simulink model "MPS_device_passive"  (R2018b)
settings: Solver=ode4  StartTime=0  StopTime=700  FixedStep=0.02  MaxStep=0.02  RelTol=1e-3  EnableMultiTasking=on
InitFcn:
  | %SSModel_calc
undefined symbols (not defined in the file): body, CentralPTOPreload, constraint, L, ML1Preload, ML2Preload, ML3Preload, ML4Preload, ML5Preload, ML6Preload, ML7Preload, ML8Preload, mrelative, pto, PTOrotation, SidePTO1Preload, SidePTO2Preload, SidePTO3Preload, SidePTO4Preload, simu, waves, X, Y, Z
libraries: nesl_utility x580, sm_lib x317, vrlib x72, WECSim_Lib x36
(part 18 of 27)

== system MPS_device_passive/PTO P3F3/VisuP3F2/Hydrodynamic Body/Wave Diffraction and Excitation Force Calculation/Linear Wave Excitation Force Variant Subsystem/Regular Wave Excitation Force ==
  note: Calculates the wave force, F_wave, for the case of Regular Waves.
      |
      | F_wave =   A * cos(w * t) * Re{Fext}
      |                -  A * sin(w * t) * Im{Fext}
  In1 : Inport
  Add : Sum
  Add1 : Sum  Inputs=+-
  Constant : Constant  Value=pi/2
  Excitation Imaginary Part : Constant  Value=body.hydroForce.fExt.im(1,:)  VectorParams1D=off
  Excitation Real Part : Constant  Value=body.hydroForce.fExt.re(1,:)  VectorParams1D=off
  Product : Product
  Product1 : Product  Inputs=3
  Product2 : Product  Inputs=3
  Sine Wave Function : Sin  TimeSource=Use external signal  SampleTime=0
  Sine Wave Function1 : Sin  TimeSource=Use external signal  SampleTime=0
  Wave Amplitude : Constant  Value=waves.A(1,:)
  Wave Frequency : Constant  Value=waves.w(1,:)
  Out1 : Outport
  wires:
  Constant/1 -> Add/2
  Add/1 -> Sine Wave Function1/1
  Wave Amplitude/1 -> Product1/1, Product2/1  "A"
  Add1/1 -> Out1/1
  Product2/1 -> Add1/2
  Product1/1 -> Add1/1
  Excitation Real Part/1 -> Product1/2  "Re{Fext}"
  Excitation Imaginary Part/1 -> Product2/3  "Im{Fext}"
  Sine Wave Function/1 -> Product2/2  "sin(wt)"
  Sine Wave Function1/1 -> Product1/3  "cos(w*t)"
  Product/1 -> Add/1, Sine Wave Function/1
  Wave Frequency/1 -> Product/2  "w"
  In1/1 -> Product/1  "t"

== system MPS_device_passive/PTO P3F3/VisuP3F2/Hydrodynamic Body/Wave Diffraction and Excitation Force Calculation/Linear Wave Excitation Force Variant Subsystem/User Defined Wave Excitation Force ==
  note: Calculates the wave force, F_wave, for the case of User Defined Waves.
      |
      | F_wave = convolution calculation [1x6]
  InputWaveForceTimeHistory : FromWorkspace  VariableName=[waves.waveAmpTime(:,1),body.hydroForce.userDefinedFe]  SampleTime=0
  Out1 : Outport
  wires:
  InputWaveForceTimeHistory/1 -> Out1/1

== system MPS_device_passive/PTO P3F3/VisuP3F2/Hydrodynamic Body/Wave Diffraction and Excitation Force Calculation/Nonlinear FK Force Variant Subsystem/No Nonlinear FroudeKrylov Force ==
  Constant : Constant  Value=[0 0 0 0 0 0]
  Out1 : Outport
  wires:
  Constant/1 -> Out1/1

== system MPS_device_passive/PTO P3F3/VisuP3F2/Hydrodynamic Body/Wave Diffraction and Excitation Force Calculation/Nonlinear FK Force Variant Subsystem/With Nonlinear FroudeKrylov Force ==
  In1 : Inport
  In2 : Inport  Port=2
  In3 : Inport  Port=3
  Add : Sum  Inputs=+-
  Center of Gravity : Constant  Value=body.hydroData.properties.cg
  Center of Gravity1 : Constant  Value=body.hydroData.properties.cg
  Constant : Constant  Value=[0 0 0]
  Deep Water Flag : Constant  Value=waves.deepWaterWave
  Diffraction and Excitation Forces : MATLAB Function  TreatAsAtomicUnit=on
  Frequency Spacing : Constant  Value=waves.dw
  Gravity : Constant  Value=simu.g
  Mux : Mux  Inputs=2
  STL Areas : Constant  Value=body.bodyGeometry.area
  STL Centers : Constant  Value=body.bodyGeometry.center
  STL Normal Vectors : Constant  Value=body.bodyGeometry.norm
  To Workspace : ToWorkspace  VariableName=body13_wavenonlinearpressure_out  SaveFormat=Structure With Time  SampleTime=-1
      settings: Decimation=round(simu.dtOut/simu.dt,0)
  To Workspace1 : ToWorkspace  VariableName=body13_wavelinearpressure_out  SaveFormat=Structure With Time  SampleTime=-1
      settings: Decimation=round(simu.dtOut/simu.dt,0)
  Water Density : Constant  Value=simu.rho
  Water Depth : Constant  Value=waves.waterDepth
  Wave Amplitude : Constant  Value=waves.A
  Wave Frequency : Constant  Value=waves.w
  Wave Number : Constant  Value=waves.k
  Wave Random Phase : Constant  Value=waves.phaseRand
  Wave Type Number : Constant  Value=waves.typeNum
  fe_calc_time : Constant  Value=simu.dtFeNonlin
  simulation_sample_time : Constant  Value=simu.dt
  Out1 : Outport
  wires:
  STL Areas/1 -> Diffraction and Excitation Forces/5(area)
  fe_calc_time/1 -> Diffraction and Excitation Forces/19(dtFe)
  simulation_sample_time/1 -> Diffraction and Excitation Forces/18(dt)
  Diffraction and Excitation Forces/2(wp) -> To Workspace/1
  Diffraction and Excitation Forces/3(wpMeanFS) -> To Workspace1/1
  In2/1 -> Add/1
  Constant/1 -> Mux/2
  Center of Gravity/1 -> Mux/1  "cg"
  Mux/1 -> Add/2
  Add/1 -> Diffraction and Excitation Forces/1(x)  "x_cg"
  Deep Water Flag/1 -> Diffraction and Excitation Forces/13(deepWaterWave)
  Wave Random Phase/1 -> Diffraction and Excitation Forces/17(phaseRand)
  Water Depth/1 -> Diffraction and Excitation Forces/12(wDepth)
  Wave Number/1 -> Diffraction and Excitation Forces/14(k)
  Wave Type Number/1 -> Diffraction and Excitation Forces/15(typeNum)
  Frequency Spacing/1 -> Diffraction and Excitation Forces/11(dw)
  Wave Frequency/1 -> Diffraction and Excitation Forces/10(w)
  Wave Amplitude/1 -> Diffraction and Excitation Forces/9(AH)
  In1/1 -> Diffraction and Excitation Forces/16(t)
  In3/1 -> Diffraction and Excitation Forces/2(elv)
  STL Centers/1 -> Diffraction and Excitation Forces/3(center)
  STL Normal Vectors/1 -> Diffraction and Excitation Forces/4(tnorm)
  Water Density/1 -> Diffraction and Excitation Forces/6(rho)
  Gravity/1 -> Diffraction and Excitation Forces/7(g)
  Diffraction and Excitation Forces/1(f) -> Out1/1
  Center of Gravity1/1 -> Diffraction and Excitation Forces/8(cg)

== system MPS_device_passive/PTO P3F3/VisuP3F2/Hydrodynamic Body/Wave Radiation Forces Calculation/SS CI and Constant-Damping-CoeVariant Subsystem/Constant Coefficients ==
  In1 : Inport
  Product : Product  Multiplication=Matrix(*)
  Radiation Damping Matrix : Constant  Value=body.hydroForce.fDamping
  Out1 : Outport
  wires:
  In1/1 -> Product/2
  Product/1 -> Out1/1  "F_Single Frequency"
  Radiation Damping Matrix/1 -> Product/1

== system MPS_device_passive/PTO P3F3/VisuP3F2/Hydrodynamic Body/Wave Radiation Forces Calculation/SS CI and Constant-Damping-CoeVariant Subsystem/Convolution Integral Calculation ==
  In1 : Inport
  In2 : Inport  Port=2
  Body-to-Body Interactions Flag : Constant  Value=body.lenJ
  Fluid Memory : MATLAB Function  TreatAsAtomicUnit=on
  Impulse Response Function K : Constant  Value=body.hydroForce.irkb
  Time (relative to the current time step) : Constant  Value=simu.CTTime  SampleTime=simu.dt
  Out1 : Outport
  wires:
  In2/1 -> Fluid Memory/5(clockTime)
  Time (relative to the current time step)/1 -> Fluid Memory/4(CTTime)
  Impulse Response Function K/1 -> Fluid Memory/3(IRKB)
  In1/1 -> Fluid Memory/2(v)
  Fluid Memory/1(F_FM) -> Out1/1  "F_Convolution Integral"
  Body-to-Body Interactions Flag/1 -> Fluid Memory/1(lenJ)

== system MPS_device_passive/PTO P3F3/VisuP3F2/Hydrodynamic Body/Wave Radiation Forces Calculation/SS CI and Constant-Damping-CoeVariant Subsystem/State-Space Calculation  ==
  In1 : Inport
  State-Space : StateSpace  A=body.hydroForce.ssRadf.A  B=body.hydroForce.ssRadf.B  C=body.hydroForce.ssRadf.C  D=body.hydroForce.ssRadf.D  InitialCondition=0
  Out1 : Outport
  wires:
  State-Space/1 -> Out1/1
  In1/1 -> State-Space/1  "x"

== system MPS_device_passive/PTO P4F4/VisuP4F1/Hydrodynamic Body/B2B Subsystem/B2B/CrossCoupling ==
  note: CrossCoupling block is updated by its mask initialization, which is only called on when a simulation is run. 'From' blocks are automatically created and connected based on the number of bodies in the simulation.
  BC1 : BusCreator  Inputs=2
  BC2 : BusCreator  Inputs=2
  vel : Outport
  acc : Outport  Port=2
  wires:
  [acc2] -> BC2/2
  [vel2] -> BC1/2
  BC2/1 -> acc/1
  BC1/1 -> vel/1
  [acc1] -> BC2/1
  [vel1] -> BC1/1

== system MPS_device_passive/PTO P4F4/VisuP4F1/Hydrodynamic Body/Hydrostatic Restoring Force Calculation/Linear and Nonlinear Restoring Force Variant Subsystem/Linear Hydrostatic Restoring Force  ==
  In1 : Inport
  Add1 : Sum  Inputs=+-
  Add2 : Sum
  Assignment (Add Net Bouyancy Force to Z-Direction) : Assignment  IndexOptions=Index vector (dialog)  Indices=3  OutputSizes=1
  Body Mass : Constant  Value=body.hydroForce.storage.mass
  Constant1 : Constant  Value=[0 0 0 0 0 0]
  Gravity : Constant  Value=simu.g
  Linear Restioring Coefficient Matrix : Constant  Value=body.hydroForce.linearHydroRestCoef
  Product : Product
  Product1 : Product  Inputs=3
  Product2 : Product  Multiplication=Matrix(*)
  Volume : Constant  Value=body.dispVol
  Water Density : Constant  Value=simu.rho
  Out1 : Outport
  wires:
  Linear Restioring Coefficient Matrix/1 -> Product2/1  "K"
  Product2/1 -> Add2/2  "Linear Restoring Force"
  Add1/1 -> Assignment (Add Net Bouyancy Force to Z-Direction)/2
  Product1/1 -> Add1/2  "F_Buoyancy"
  Product/1 -> Add1/1  "F_Gravity"
  Water Density/1 -> Product1/1  "rho"
  Gravity/1 -> Product/1, Product1/2  "g"
  Volume/1 -> Product1/3  "Vol"
  Add2/1 -> Out1/1  "F_Restoring"
  Assignment (Add Net Bouyancy Force to Z-Direction)/1 -> Add2/1  "Net Buoyancy Force"
  Constant1/1 -> Assignment (Add Net Bouyancy Force to Z-Direction)/1
  Body Mass/1 -> Product/2  "m"
  In1/1 -> Product2/2  "x"

== system MPS_device_passive/PTO P4F4/VisuP4F1/Hydrodynamic Body/Hydrostatic Restoring Force Calculation/Linear and Nonlinear Restoring Force Variant Subsystem/Nonlinear Hydrostatic Restoring Force ==
  In1 : Inport
  In2 : Inport  Port=2
  In3 : Inport  Port=3
  Add3 : Sum  Inputs=-+
  Assignment (Add Net Bouyancy Force to Z-Direction)2 : Assignment  IndexOptions=Index vector (dialog)  Indices=3  OutputSizes=1
  Body Mass1 : Constant  Value=body.hydroForce.storage.mass
  Center of Gravity : Constant  Value=body.cg
  Constant2 : Constant  Value=[0 0 0 0 0 0]
  Diffarction and Excitation Forces1 : MATLAB Function  TreatAsAtomicUnit=on
  Gravity2 : Constant  Value=simu.g
  Product3 : Product
  SImulation Step Time : Constant  Value=simu.dt
  STL areas : Constant  Value=body.bodyGeometry.area
  STL centers : Constant  Value=body.bodyGeometry.center
  STL normal vectors : Constant  Value=body.bodyGeometry.norm
  Simulation Fe Calc Step Time : Constant  Value=simu.dtFeNonlin
  To Workspace1 : ToWorkspace  VariableName=body16_hspressure_out  SaveFormat=Structure With Time  SampleTime=-1
      settings: Decimation=round(simu.dtOut/simu.dt,0)
  Water Density1 : Constant  Value=simu.rho
  Out1 : Outport
  wires:
  STL areas/1 -> Diffarction and Excitation Forces1/5(area)
  In3/1 -> Diffarction and Excitation Forces1/11(t)
  Simulation Fe Calc Step Time/1 -> Diffarction and Excitation Forces1/10(dtFe)
  SImulation Step Time/1 -> Diffarction and Excitation Forces1/9(dt)
  Diffarction and Excitation Forces1/2(p) -> To Workspace1/1
  In2/1 -> Diffarction and Excitation Forces1/2(elv)
  STL centers/1 -> Diffarction and Excitation Forces1/3(center)
  STL normal vectors/1 -> Diffarction and Excitation Forces1/4(tnorm)
  Water Density1/1 -> Diffarction and Excitation Forces1/6(rho)
  Gravity2/1 -> Diffarction and Excitation Forces1/7(g), Product3/1  "g"
  Body Mass1/1 -> Product3/2
  Constant2/1 -> Assignment (Add Net Bouyancy Force to Z-Direction)2/1
  Product3/1 -> Assignment (Add Net Bouyancy Force to Z-Direction)2/2
  Diffarction and Excitation Forces1/1(f) -> Add3/1
  Add3/1 -> Out1/1
  Assignment (Add Net Bouyancy Force to Z-Direction)2/1 -> Add3/2
  Center of Gravity/1 -> Diffarction and Excitation Forces1/8(cg)
  In1/1 -> Diffarction and Excitation Forces1/1(x)

== system MPS_device_passive/PTO P4F4/VisuP4F1/Hydrodynamic Body/Morrison Element and ViscousDampingForceCalculation/Morrison Element Variant Subsystem/Morrison Element Off ==
  Constant : Constant  Value=[0 0 0 0 0 0]
  morison_force : Outport
  wires:
  Constant/1 -> morison_force/1

== system MPS_device_passive/PTO P4F4/VisuP4F1/Hydrodynamic Body/Morrison Element and ViscousDampingForceCalculation/Morrison Element Variant Subsystem/Morrison Element On ==
  note: 1) Add Subsystem or Model blocks as valid variant choices.
      | 2) You cannot connect blocks at this level. At simulation, connectivity is automatically
      | determined, based on the active variant and port name matching.
  displacement : Inport
  velocity : Inport  Port=2
  acceleration : Inport  Port=3
  time : Inport  Port=4
  Irregular Wave Morison Force : Subsystem  VariantControl=sv_irregularWaves
  No Wave Morison Force : Subsystem  VariantControl=sv_noWave
  Regular Wave Morison Force : Subsystem  VariantControl=sv_regularWaves
  morison_force : Outport

== system MPS_device_passive/PTO P4F4/VisuP4F1/Hydrodynamic Body/Nonlinear Wave Elevation/Linear or Instantaneous Free Surface/Instantaneous Water Free Surface   ==
  In1 : Inport
  In2 : Inport  Port=2
  Center of Gravity : Constant  Value=body.cg
  Frequency Spacing : Constant  Value=waves.dw
  Instantaneous FS : MATLAB Function  TreatAsAtomicUnit=on
  Ramp Time : Constant  Value=simu.rampT
  STL Centers : Constant  Value=body.bodyGeometry.center
  Simulation Time Step : Constant  Value=simu.dt
  Time Step for Non-Linear Forces : Constant  Value=simu.dtFeNonlin
  Wave Amplitude : Constant  Value=waves.A
  Wave Direction : Constant  Value=waves.waveDir
  Wave Frequency : Constant  Value=waves.w
  Wave Number : Constant  Value=waves.k
  Wave Random Phase : Constant  Value=waves.phaseRand
  Wave Type Number : Constant  Value=waves.typeNum
  Out1 : Outport
  wires:
  Wave Amplitude/1 -> Instantaneous FS/4(AH)
  Time Step for Non-Linear Forces/1 -> Instantaneous FS/14(dtFe)
  Simulation Time Step/1 -> Instantaneous FS/13(dt)
  Wave Direction/1 -> Instantaneous FS/12(waveDir)
  In1/1 -> Instantaneous FS/1(x)
  In2/1 -> Instantaneous FS/9(t)
  Frequency Spacing/1 -> Instantaneous FS/6(dw)
  Wave Random Phase/1 -> Instantaneous FS/11(phaseRand)
  Ramp Time/1 -> Instantaneous FS/10(rampT)
  Wave Type Number/1 -> Instantaneous FS/8(typeNum)
  Wave Frequency/1 -> Instantaneous FS/5(w)
  Wave Number/1 -> Instantaneous FS/7(k)
  Center of Gravity/1 -> Instantaneous FS/3(cg)
  STL Centers/1 -> Instantaneous FS/2(center)
  Instantaneous FS/1(f) -> Out1/1

== system MPS_device_passive/PTO P4F4/VisuP4F1/Hydrodynamic Body/Nonlinear Wave Elevation/Linear or Instantaneous Free Surface/Mean Water Free Surface  ==
  zero : Constant  Value=0
  Out1 : Outport
  wires:
  zero/1 -> Out1/1

== system MPS_device_passive/PTO P4F4/VisuP4F1/Hydrodynamic Body/Wave Diffraction and Excitation Force Calculation/Linear Wave Excitation Force Variant Subsystem/Irregular Wave Excitation Force ==
  note: Calculates the wave force, F_wave, for the case of Irregular Waves.
      |
      | F_wave = sum( F_wave(i))
      |
      | where i = each frequency bin.
  In1 : Inport
  Frequency Spacing Delta Omega : Constant  Value=waves.dw  VectorParams1D=off
  Imaginary Part of Wave Excitation : Constant  Value=body.hydroForce.fExt.im  VectorParams1D=off
  MATLAB Function : MATLAB Function  TreatAsAtomicUnit=on
  Random Phase : Constant  Value=waves.phaseRand  VectorParams1D=off
  Real Part of Wave Excitation : Constant  Value=body.hydroForce.fExt.re  VectorParams1D=off
  Wave Frequency : Constant  Value=waves.w  VectorParams1D=off
  Wave Spectrum : Constant  Value=waves.A  VectorParams1D=off
  Out1 : Outport
  wires:
  Frequency Spacing Delta Omega/1 -> MATLAB Function/6(dw)
  In1/1 -> MATLAB Function/7(time)
  Wave Spectrum/1 -> MATLAB Function/1(A)
  Real Part of Wave Excitation/1 -> MATLAB Function/3(fExtRE)
  Imaginary Part of Wave Excitation/1 -> MATLAB Function/4(fExtIM)
  Wave Frequency/1 -> MATLAB Function/2(w)
  MATLAB Function/1(Fext) -> Out1/1
  Random Phase/1 -> MATLAB Function/5(phaseRand)

== system MPS_device_passive/PTO P4F4/VisuP4F1/Hydrodynamic Body/Wave Diffraction and Excitation Force Calculation/Linear Wave Excitation Force Variant Subsystem/No Wave Excitation Force ==
  Constant : Constant  Value=[0 0 0 0 0 0]
  Out1 : Outport
  wires:
  Constant/1 -> Out1/1

== system MPS_device_passive/PTO P4F4/VisuP4F1/Hydrodynamic Body/Wave Diffraction and Excitation Force Calculation/Linear Wave Excitation Force Variant Subsystem/Regular Wave Excitation Force ==
  note: Calculates the wave force, F_wave, for the case of Regular Waves.
      |
      | F_wave =   A * cos(w * t) * Re{Fext}
      |                -  A * sin(w * t) * Im{Fext}
  In1 : Inport
  Add : Sum
  Add1 : Sum  Inputs=+-
  Constant : Constant  Value=pi/2
  Excitation Imaginary Part : Constant  Value=body.hydroForce.fExt.im(1,:)  VectorParams1D=off
  Excitation Real Part : Constant  Value=body.hydroForce.fExt.re(1,:)  VectorParams1D=off
  Product : Product
  Product1 : Product  Inputs=3
  Product2 : Product  Inputs=3
  Sine Wave Function : Sin  TimeSource=Use external signal  SampleTime=0
  Sine Wave Function1 : Sin  TimeSource=Use external signal  SampleTime=0
  Wave Amplitude : Constant  Value=waves.A(1,:)
  Wave Frequency : Constant  Value=waves.w(1,:)
  Out1 : Outport
  wires:
  Constant/1 -> Add/2
  Add/1 -> Sine Wave Function1/1
  Wave Amplitude/1 -> Product1/1, Product2/1  "A"
  Add1/1 -> Out1/1
  Product2/1 -> Add1/2
  Product1/1 -> Add1/1
  Excitation Real Part/1 -> Product1/2  "Re{Fext}"
  Excitation Imaginary Part/1 -> Product2/3  "Im{Fext}"
  Sine Wave Function/1 -> Product2/2  "sin(wt)"
  Sine Wave Function1/1 -> Product1/3  "cos(w*t)"
  Product/1 -> Add/1, Sine Wave Function/1
  Wave Frequency/1 -> Product/2  "w"
  In1/1 -> Product/1  "t"

== system MPS_device_passive/PTO P4F4/VisuP4F1/Hydrodynamic Body/Wave Diffraction and Excitation Force Calculation/Linear Wave Excitation Force Variant Subsystem/User Defined Wave Excitation Force ==
  note: Calculates the wave force, F_wave, for the case of User Defined Waves.
      |
      | F_wave = convolution calculation [1x6]
  InputWaveForceTimeHistory : FromWorkspace  VariableName=[waves.waveAmpTime(:,1),body.hydroForce.userDefinedFe]  SampleTime=0
  Out1 : Outport
  wires:
  InputWaveForceTimeHistory/1 -> Out1/1

== system MPS_device_passive/PTO P4F4/VisuP4F1/Hydrodynamic Body/Wave Diffraction and Excitation Force Calculation/Nonlinear FK Force Variant Subsystem/No Nonlinear FroudeKrylov Force ==
  Constant : Constant  Value=[0 0 0 0 0 0]
  Out1 : Outport
  wires:
  Constant/1 -> Out1/1

== system MPS_device_passive/PTO P4F4/VisuP4F1/Hydrodynamic Body/Wave Diffraction and Excitation Force Calculation/Nonlinear FK Force Variant Subsystem/With Nonlinear FroudeKrylov Force ==
  In1 : Inport
  In2 : Inport  Port=2
  In3 : Inport  Port=3
  Add : Sum  Inputs=+-
  Center of Gravity : Constant  Value=body.hydroData.properties.cg
  Center of Gravity1 : Constant  Value=body.hydroData.properties.cg
  Constant : Constant  Value=[0 0 0]
  Deep Water Flag : Constant  Value=waves.deepWaterWave
  Diffraction and Excitation Forces : MATLAB Function  TreatAsAtomicUnit=on
  Frequency Spacing : Constant  Value=waves.dw
  Gravity : Constant  Value=simu.g
  Mux : Mux  Inputs=2
  STL Areas : Constant  Value=body.bodyGeometry.area
  STL Centers : Constant  Value=body.bodyGeometry.center
  STL Normal Vectors : Constant  Value=body.bodyGeometry.norm
  To Workspace : ToWorkspace  VariableName=body16_wavenonlinearpressure_out  SaveFormat=Structure With Time  SampleTime=-1
      settings: Decimation=round(simu.dtOut/simu.dt,0)
  To Workspace1 : ToWorkspace  VariableName=body16_wavelinearpressure_out  SaveFormat=Structure With Time  SampleTime=-1
      settings: Decimation=round(simu.dtOut/simu.dt,0)
  Water Density : Constant  Value=simu.rho
  Water Depth : Constant  Value=waves.waterDepth
  Wave Amplitude : Constant  Value=waves.A
  Wave Frequency : Constant  Value=waves.w
  Wave Number : Constant  Value=waves.k
  Wave Random Phase : Constant  Value=waves.phaseRand
  Wave Type Number : Constant  Value=waves.typeNum
  fe_calc_time : Constant  Value=simu.dtFeNonlin
  simulation_sample_time : Constant  Value=simu.dt
  Out1 : Outport
  wires:
  STL Areas/1 -> Diffraction and Excitation Forces/5(area)
  fe_calc_time/1 -> Diffraction and Excitation Forces/19(dtFe)
  simulation_sample_time/1 -> Diffraction and Excitation Forces/18(dt)
  Diffraction and Excitation Forces/2(wp) -> To Workspace/1
  Diffraction and Excitation Forces/3(wpMeanFS) -> To Workspace1/1
  In2/1 -> Add/1
  Constant/1 -> Mux/2
  Center of Gravity/1 -> Mux/1  "cg"
  Mux/1 -> Add/2
  Add/1 -> Diffraction and Excitation Forces/1(x)  "x_cg"
  Deep Water Flag/1 -> Diffraction and Excitation Forces/13(deepWaterWave)
  Wave Random Phase/1 -> Diffraction and Excitation Forces/17(phaseRand)
  Water Depth/1 -> Diffraction and Excitation Forces/12(wDepth)
  Wave Number/1 -> Diffraction and Excitation Forces/14(k)
  Wave Type Number/1 -> Diffraction and Excitation Forces/15(typeNum)
  Frequency Spacing/1 -> Diffraction and Excitation Forces/11(dw)
  Wave Frequency/1 -> Diffraction and Excitation Forces/10(w)
  Wave Amplitude/1 -> Diffraction and Excitation Forces/9(AH)
  In1/1 -> Diffraction and Excitation Forces/16(t)
  In3/1 -> Diffraction and Excitation Forces/2(elv)
  STL Centers/1 -> Diffraction and Excitation Forces/3(center)
  STL Normal Vectors/1 -> Diffraction and Excitation Forces/4(tnorm)
  Water Density/1 -> Diffraction and Excitation Forces/6(rho)
  Gravity/1 -> Diffraction and Excitation Forces/7(g)
  Diffraction and Excitation Forces/1(f) -> Out1/1
  Center of Gravity1/1 -> Diffraction and Excitation Forces/8(cg)

== system MPS_device_passive/PTO P4F4/VisuP4F1/Hydrodynamic Body/Wave Radiation Forces Calculation/SS CI and Constant-Damping-CoeVariant Subsystem/Constant Coefficients ==
  In1 : Inport
  Product : Product  Multiplication=Matrix(*)
  Radiation Damping Matrix : Constant  Value=body.hydroForce.fDamping
  Out1 : Outport
  wires:
  In1/1 -> Product/2
  Product/1 -> Out1/1  "F_Single Frequency"
  Radiation Damping Matrix/1 -> Product/1

== system MPS_device_passive/PTO P4F4/VisuP4F1/Hydrodynamic Body/Wave Radiation Forces Calculation/SS CI and Constant-Damping-CoeVariant Subsystem/Convolution Integral Calculation ==
  In1 : Inport
  In2 : Inport  Port=2
  Body-to-Body Interactions Flag : Constant  Value=body.lenJ
  Fluid Memory : MATLAB Function  TreatAsAtomicUnit=on
  Impulse Response Function K : Constant  Value=body.hydroForce.irkb
  Time (relative to the current time step) : Constant  Value=simu.CTTime  SampleTime=simu.dt
  Out1 : Outport
  wires:
  In2/1 -> Fluid Memory/5(clockTime)
  Time (relative to the current time step)/1 -> Fluid Memory/4(CTTime)
  Impulse Response Function K/1 -> Fluid Memory/3(IRKB)
  In1/1 -> Fluid Memory/2(v)
  Fluid Memory/1(F_FM) -> Out1/1  "F_Convolution Integral"
  Body-to-Body Interactions Flag/1 -> Fluid Memory/1(lenJ)

== system MPS_device_passive/PTO P4F4/VisuP4F1/Hydrodynamic Body/Wave Radiation Forces Calculation/SS CI and Constant-Damping-CoeVariant Subsystem/State-Space Calculation  ==
  In1 : Inport
  State-Space : StateSpace  A=body.hydroForce.ssRadf.A  B=body.hydroForce.ssRadf.B  C=body.hydroForce.ssRadf.C  D=body.hydroForce.ssRadf.D  InitialCondition=0
  Out1 : Outport
  wires:
  State-Space/1 -> Out1/1
  In1/1 -> State-Space/1  "x"

== system MPS_device_passive/Reactor/Hydrodynamic Body/Morrison Element and ViscousDampingForceCalculation/Morrison Element Variant Subsystem/Morrison Element On/Irregular Wave Excitation Force ==
  In1 : Inport
  In2 : Inport  Port=2
  In3 : Inport  Port=3
  In4 : Inport  Port=4
  Area : Constant  Value=body.morrisonElement.characteristicArea  VectorParams1D=off
  Ca : Constant  Value=body.morrisonElement.ca  VectorParams1D=off
  Cd : Constant  Value=body.morrisonElement.cd  VectorParams1D=off
  MESum : Sum  Inputs=+  CollapseMode=Specified dimension
  MorrisonElements : Subsystem  TreatAsAtomicUnit=on
  Reshape : Reshape
  Volume : Constant  Value=body.morrisonElement.VME  VectorParams1D=off
  "r_{g}" : Constant  Value=body.morrisonElement.rgME  VectorParams1D=off
  Out1 : Outport
  wires:
  In4/1 -> MorrisonElements/9(Time)
  MESum/1 -> Reshape/1
  Reshape/1 -> Out1/1
  MorrisonElements/1(Force) -> MESum/1
  Ca/1 -> MorrisonElements/8(Ca)
  Volume/1 -> MorrisonElements/7(Vol)
  In3/1 -> MorrisonElements/3(Accel)
  In1/1 -> MorrisonElements/4(Disp)
  Cd/1 -> MorrisonElements/6(Cd)
  Area/1 -> MorrisonElements/5(A)
  "r_{g}"/1 -> MorrisonElements/1(r)
  In2/1 -> MorrisonElements/2(Vel)

== system MPS_device_passive/Reactor/Hydrodynamic Body/Morrison Element and ViscousDampingForceCalculation/Morrison Element Variant Subsystem/Morrison Element On/No Wave Excitation Force ==
  In1 : Inport
  In2 : Inport  Port=2
  In3 : Inport  Port=3
  In4 : Inport  Port=4
  Area : Constant  Value=body.morrisonElement.characteristicArea  VectorParams1D=off
  Ca : Constant  Value=body.morrisonElement.ca  VectorParams1D=off
  Cd : Constant  Value=body.morrisonElement.cd  VectorParams1D=off
  MESum : Sum  Inputs=+  CollapseMode=Specified dimension
  MorrisonElements : Subsystem  TreatAsAtomicUnit=on
  Reshape : Reshape
  Volume : Constant  Value=body.morrisonElement.VME  VectorParams1D=off
  "r_{g}" : Constant  Value=body.morrisonElement.rgME  VectorParams1D=off
  Out1 : Outport
  wires:
  In4/1 -> MorrisonElements/9(Time)
  Reshape/1 -> Out1/1
  MESum/1 -> Reshape/1
  In3/1 -> MorrisonElements/3(Accel)
  In2/1 -> MorrisonElements/2(Vel)
  In1/1 -> MorrisonElements/4(Disp)
  Ca/1 -> MorrisonElements/8(Ca)
  Volume/1 -> MorrisonElements/7(Vol)
  MorrisonElements/1(Force) -> MESum/1
  Cd/1 -> MorrisonElements/6(Cd)
  Area/1 -> MorrisonElements/5(Area)
  "r_{g}"/1 -> MorrisonElements/1(r)

== system MPS_device_passive/Reactor/Hydrodynamic Body/Morrison Element and ViscousDampingForceCalculation/Morrison Element Variant Subsystem/Morrison Element On/Regular Wave Excitation Force ==
  In1 : Inport
  In2 : Inport  Port=2
  In3 : Inport  Port=3
  In4 : Inport  Port=4
  Area : Constant  Value=body.morrisonElement.characteristicArea  VectorParams1D=off
  Ca : Constant  Value=body.morrisonElement.ca  VectorParams1D=off
  Cd : Constant  Value=body.morrisonElement.cd  VectorParams1D=off
  MESum : Sum  Inputs=+  CollapseMode=Specified dimension
  MorrisonElements : Subsystem  TreatAsAtomicUnit=on
  Reshape : Reshape
  Volume : Constant  Value=body.morrisonElement.VME  VectorParams1D=off
  "r_{g}" : Constant  Value=body.morrisonElement.rgME  VectorParams1D=off
  Out1 : Outport
  wires:
  In4/1 -> MorrisonElements/9(Time)
  Reshape/1 -> Out1/1
  MESum/1 -> Reshape/1
  In3/1 -> MorrisonElements/3(Accel)
  In2/1 -> MorrisonElements/2(Vel)
  In1/1 -> MorrisonElements/4(Disp)
  Ca/1 -> MorrisonElements/8(Ca)
  Volume/1 -> MorrisonElements/7(Vol)
  MorrisonElements/1(Force) -> MESum/1
  Cd/1 -> MorrisonElements/6(Cd)
  Area/1 -> MorrisonElements/5(Area)
  "r_{g}"/1 -> MorrisonElements/1(r)

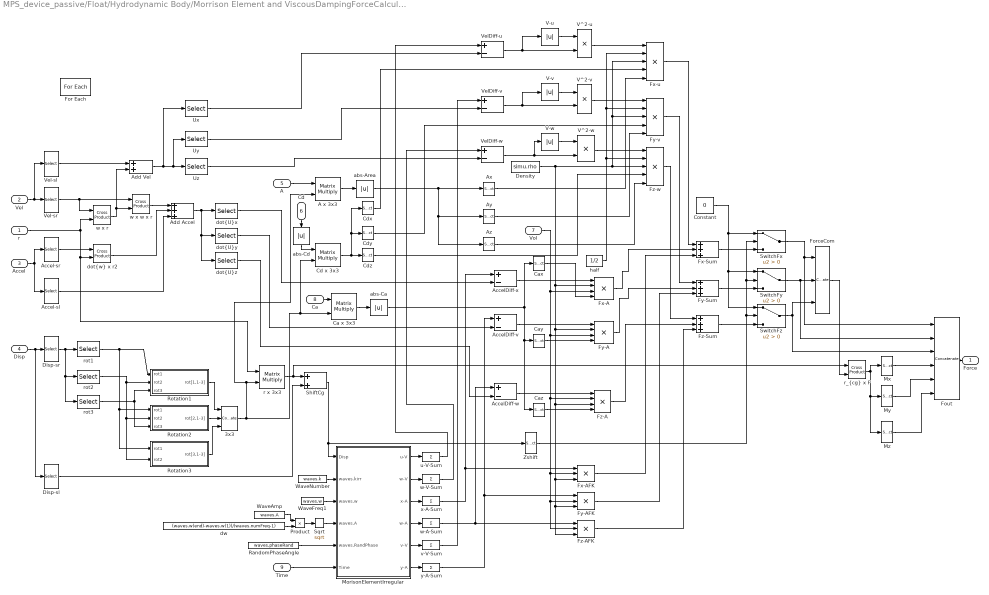
== system MPS_device_passive/Float/Hydrodynamic Body/Morrison Element and ViscousDampingForceCalculation/Morrison Element Variant Subsystem/Morrison Element On/Irregular Wave Morison Force/MorrisonElements ==
  r : Inport  Partition=on  PartitionDimension=1  PartitionWidth=1  PartitionOffset=0
  Vel : Inport  Port=2
  Accel : Inport  Port=3
  Disp : Inport  Port=4
  A : Inport  Port=5  Partition=on  PartitionDimension=1  PartitionWidth=1  PartitionOffset=0
  Cd : Inport  Port=6  Partition=on  PartitionDimension=1  PartitionWidth=1  PartitionOffset=0
  Vol : Inport  Port=7  Partition=on  PartitionDimension=1  PartitionWidth=1  PartitionOffset=0
  Ca : Inport  Port=8  Partition=on  PartitionDimension=1  PartitionWidth=1  PartitionOffset=0
  Time : Inport  Port=9
  3x3 : Concatenate  NumInputs=3  Mode=Multidimensional array
  A x 3x3 : Product  Multiplication=Matrix(*)
  Accel-sl : Selector  InputPortWidth=6  IndexOptions=Index vector (dialog)  Indices=[1 2 3]  OutputSizes=1
  Accel-sr : Selector  InputPortWidth=6  IndexOptions=Index vector (dialog)  Indices=[4 5 6]  OutputSizes=1
  AccelDiff-v : Sum  Inputs=+-
  AccelDiff-w : Sum  Inputs=+-
  AccelDiff-x : Sum  Inputs=+-
  Add Accel : Sum  Inputs=+++
  Add Vel : Sum
  Ax : Selector  InputPortWidth=3  IndexOptions=Index vector (dialog)  Indices=[1]  OutputSizes=1
  Ay : Selector  InputPortWidth=3  IndexOptions=Index vector (dialog)  Indices=[2]  OutputSizes=1
  Az : Selector  InputPortWidth=3  IndexOptions=Index vector (dialog)  Indices=[3]  OutputSizes=1
  Ca x 3x3 : Product  Multiplication=Matrix(*)
  Cax : Selector  InputPortWidth=3  IndexOptions=Index vector (dialog)  Indices=[1]  OutputSizes=1
  Cay : Selector  InputPortWidth=3  IndexOptions=Index vector (dialog)  Indices=[2]  OutputSizes=1
  Caz : Selector  InputPortWidth=3  IndexOptions=Index vector (dialog)  Indices=[3]  OutputSizes=1
  Cd x 3x3 : Product  Multiplication=Matrix(*)
  Cdx : Selector  InputPortWidth=3  IndexOptions=Index vector (dialog)  Indices=[1]  OutputSizes=1
  Cdy : Selector  InputPortWidth=3  IndexOptions=Index vector (dialog)  Indices=[2]  OutputSizes=1
  Cdz : Selector  InputPortWidth=3  IndexOptions=Index vector (dialog)  Indices=[3]  OutputSizes=1
  Constant : Constant  Value=0
  Density : Constant  Value=simu.rho
  Disp-sl : Selector  InputPortWidth=6  IndexOptions=Index vector (dialog)  Indices=[1 2 3]  OutputSizes=1
  Disp-sr : Selector  InputPortWidth=6  IndexOptions=Index vector (dialog)  Indices=[4 5 6]  OutputSizes=1
  For Each : ForEach  DisableCoverage=on  IndexMode=One-based
  ForceCom : Concatenate  NumInputs=3  ConcatenateDimension=2
  Fout : Concatenate  NumInputs=6  Mode=Multidimensional array  ConcatenateDimension=2
  Fx-A : Product  Inputs=4
  Fx-AFK : Product  Inputs=3
  Fx-Sum : Sum  Inputs=+++
  Fx-u : Product  Inputs=5
  Fy-A : Product  Inputs=4
  Fy-AFK : Product  Inputs=3
  Fy-Sum : Sum  Inputs=+++
  Fy-v : Product  Inputs=5
  Fz-A : Product  Inputs=4
  Fz-AFK : Product  Inputs=3
  Fz-Sum : Sum  Inputs=+++
  Fz-w : Product  Inputs=5
  MorisonElementIrregular : Subsystem  TreatAsAtomicUnit=on
  Mx : Selector  InputPortWidth=3  IndexOptions=Index vector (dialog)  Indices=[1]  OutputSizes=1
  My : Selector  InputPortWidth=3  IndexOptions=Index vector (dialog)  Indices=[2]  OutputSizes=1
  Mz : Selector  InputPortWidth=3  IndexOptions=Index vector (dialog)  Indices=[3]  OutputSizes=1
  Product : Product
  RandomPhaseAngle : Constant  Value=waves.phaseRand  VectorParams1D=off
  Rotation1 : Subsystem
  Rotation2 : Subsystem
  Rotation3 : Subsystem
  ShiftCg : Sum
  Sqrt : Sqrt  SaturateOnIntegerOverflow=on
  SwitchFx : Switch  Criteria=u2 > Threshold
  SwitchFy : Switch  Criteria=u2 > Threshold
  SwitchFz : Switch  Criteria=u2 > Threshold
  Ux : Selector  InputPortWidth=3  IndexOptions=Index vector (dialog)  Indices=[1]  OutputSizes=1
  Uy : Selector  InputPortWidth=3  IndexOptions=Index vector (dialog)  Indices=[2]  OutputSizes=1
  Uz : Selector  InputPortWidth=3  IndexOptions=Index vector (dialog)  Indices=[3]  OutputSizes=1
  V-u : Abs
  V-v : Abs
  V-w : Abs
  V^2-u : Product
  V^2-v : Product
  V^2-w : Product
  Vel-sl : Selector  InputPortWidth=6  IndexOptions=Index vector (dialog)  Indices=[1 2 3]  OutputSizes=1
  "Vel-sr " : Selector  InputPortWidth=6  IndexOptions=Index vector (dialog)  Indices=[4 5 6]  OutputSizes=1
  VelDiff-u : Sum  Inputs=+-
  VelDiff-v : Sum  Inputs=+-
  VelDiff-w : Sum  Inputs=+-
  WaveAmp : Constant  Value=waves.A  VectorParams1D=off
  WaveFreq1 : Constant  Value=waves.w  VectorParams1D=off
  WaveNumber : Constant  Value=waves.k  VectorParams1D=off
  Zshift : Selector  InputPortWidth=3  IndexOptions=Index vector (dialog)  Indices=[3]  OutputSizes=1
  abs-Area : Abs
  abs-Ca : Abs
  abs-Cd : Abs
  "dot{U}x" : Selector  InputPortWidth=3  IndexOptions=Index vector (dialog)  Indices=[1]  OutputSizes=1
  "dot{U}y" : Selector  InputPortWidth=3  IndexOptions=Index vector (dialog)  Indices=[2]  OutputSizes=1
  "dot{U}z" : Selector  InputPortWidth=3  IndexOptions=Index vector (dialog)  Indices=[3]  OutputSizes=1
  "dot{w} x r2" : vrlib/Utilities/Cross Product
      settings: SourceProductBaseCode=VR
  dw : Constant  Value=(waves.w(end)-waves.w(1))/(waves.numFreq-1)  VectorParams1D=off
  half : Constant  Value=1/2
  r x 3x3 : Product  Multiplication=Matrix(*)
  "r_{cg} x F" : vrlib/Utilities/Cross Product
      settings: SourceProductBaseCode=VR
  rot1 : Selector  InputPortWidth=3  IndexOptions=Index vector (dialog)  Indices=[1]  OutputSizes=1
  rot2 : Selector  InputPortWidth=3  IndexOptions=Index vector (dialog)  Indices=[2]  OutputSizes=1
  rot3 : Selector  InputPortWidth=3  IndexOptions=Index vector (dialog)  Indices=[3]  OutputSizes=1
  u-V-Sum : Sum  Inputs=+  CollapseMode=Specified dimension
  v-V-Sum : Sum  Inputs=+  CollapseMode=Specified dimension
  w x r : vrlib/Utilities/Cross Product
      settings: SourceProductBaseCode=VR
  w x w x r : vrlib/Utilities/Cross Product
      settings: SourceProductBaseCode=VR
  w-A-Sum : Sum  Inputs=+  CollapseMode=Specified dimension
  w-V-Sum : Sum  Inputs=+  CollapseMode=Specified dimension
  x-A-Sum : Sum  Inputs=+  CollapseMode=Specified dimension
  y-A-Sum : Sum  Inputs=+  CollapseMode=Specified dimension
  Force : Outport  PortDimensions=[1 6]  ConcatenationDimension=1
  wires:
  Time/1 -> MorisonElementIrregular/6(Time)
  abs-Cd/1 -> Cd x 3x3/1
  abs-Ca/1 -> Cay/1, Caz/1, Cax/1
  Fy-AFK/1 -> Fy-Sum/3
  Fy-A/1 -> Fy-Sum/2
  AccelDiff-v/1 -> Fy-A/1
  Cay/1 -> Fy-A/4
  y-A-Sum/1 -> AccelDiff-v/1, Fy-AFK/1
  Fy-v/1 -> Fy-Sum/1
  Fy-Sum/1 -> SwitchFy/3
  SwitchFy/1 -> ForceCom/2, Fout/2
  Cdy/1 -> Fy-v/4
  Ay/1 -> Fy-v/5
  V^2-v/1 -> Fy-v/1
  v-V-Sum/1 -> VelDiff-v/1
  V-v/1 -> V^2-v/1
  VelDiff-v/1 -> V^2-v/2, V-v/1
  V-w/1 -> V^2-w/1
  MorisonElementIrregular/6(y-A) -> y-A-Sum/1
  MorisonElementIrregular/5(v-V) -> v-V-Sum/1
  V-u/1 -> V^2-u/1
  MorisonElementIrregular/4(w-A) -> w-A-Sum/1
  MorisonElementIrregular/3(x-A) -> x-A-Sum/1
  MorisonElementIrregular/2(w-V) -> w-V-Sum/1
  Sqrt/1 -> MorisonElementIrregular/4(waves.A)
  Product/1 -> Sqrt/1
  dw/1 -> Product/2
  WaveAmp/1 -> Product/1
  MorisonElementIrregular/1(u-V) -> u-V-Sum/1
  RandomPhaseAngle/1 -> MorisonElementIrregular/5(waves.RandPhase)
  WaveFreq1/1 -> MorisonElementIrregular/3(waves.w)
  WaveNumber/1 -> MorisonElementIrregular/2(waves.kirr)
  Ca x 3x3/1 -> abs-Ca/1
  Ca/1 -> Ca x 3x3/1
  Cd x 3x3/1 -> Cdx/1, Cdy/1, Cdz/1
  Cd/1 -> abs-Cd/1
  Cax/1 -> Fx-A/4
  Caz/1 -> Fz-A/4
  Fout/1 -> Force/1
  ForceCom/1 -> "r_{cg} x F"/2
  abs-Area/1 -> Ax/1, Az/1, Ay/1
  A x 3x3/1 -> abs-Area/1
  Cdz/1 -> Fz-w/4
  Cdx/1 -> Fx-u/4
  Ax/1 -> Fx-u/5
  A/1 -> A x 3x3/1
  Az/1 -> Fz-w/5
  Fz-Sum/1 -> SwitchFz/3
  Fx-Sum/1 -> SwitchFx/3
  SwitchFx/1 -> ForceCom/1, Fout/1
  SwitchFz/1 -> Fout/3, ForceCom/3
  Zshift/1 -> SwitchFz/2, SwitchFx/2, SwitchFy/2
  VelDiff-u/1 -> V^2-u/2, V-u/1
  3x3/1 -> Cd x 3x3/2, Ca x 3x3/2, r x 3x3/2, A x 3x3/2
  Mz/1 -> Fout/6
  My/1 -> Fout/5
  Mx/1 -> Fout/4
  "r_{cg} x F"/1 -> Mx/1, My/1, Mz/1
  Constant/1 -> SwitchFx/1, SwitchFz/1, SwitchFy/1
  Fz-AFK/1 -> Fz-Sum/3
  Fz-A/1 -> Fz-Sum/2
  Fz-w/1 -> Fz-Sum/1
  Fx-AFK/1 -> Fx-Sum/3
  Fx-A/1 -> Fx-Sum/2
  Fx-u/1 -> Fx-Sum/1
  w-A-Sum/1 -> Fz-AFK/1, AccelDiff-w/1
  AccelDiff-w/1 -> Fz-A/1
  Vol/1 -> Fx-A/3, Fz-A/2, Fx-AFK/2, Fz-AFK/2, Fy-AFK/2, Fy-A/3
  AccelDiff-x/1 -> Fx-A/1
  V^2-w/1 -> Fz-w/1
  Density/1 -> Fz-w/3, Fx-u/3, Fy-v/3, Fx-A/2, Fz-A/3, Fx-AFK/3, Fz-AFK/3, Fy-AFK/3, Fy-A/2
  half/1 -> Fx-u/2, Fy-v/2, Fz-w/2
  V^2-u/1 -> Fx-u/1
  VelDiff-w/1 -> V-w/1, V^2-w/2
  w-V-Sum/1 -> VelDiff-w/1
  u-V-Sum/1 -> VelDiff-u/1
  Uz/1 -> VelDiff-w/2
  Ux/1 -> VelDiff-u/2
  Uy/1 -> VelDiff-v/2
  Add Vel/1 -> Uz/1, Uy/1, Ux/1
  "dot{U}z"/1 -> AccelDiff-w/2
  x-A-Sum/1 -> AccelDiff-x/1, Fx-AFK/1
  "dot{U}x"/1 -> AccelDiff-x/2
  "dot{U}y"/1 -> AccelDiff-v/2
  ShiftCg/1 -> Zshift/1, MorisonElementIrregular/1(Disp)
  Disp-sl/1 -> ShiftCg/2
  r x 3x3/1 -> ShiftCg/1, "r_{cg} x F"/1
  Rotation3/1(rot[3,1-3]) -> 3x3/3
  Rotation1/1(rot[1,1-3]) -> 3x3/1
  Rotation2/1(rot[2,1-3]) -> 3x3/2
  rot2/1 -> Rotation1/2(rot2), Rotation2/2(rot2), Rotation3/2(rot2)
  rot1/1 -> Rotation1/1(rot1), Rotation2/1(rot1), Rotation3/1(rot1)
  rot3/1 -> Rotation1/3(rot3), Rotation2/3(rot3)
  Disp-sr/1 -> rot1/1, rot2/1, rot3/1
  Disp/1 -> Disp-sr/1, Disp-sl/1
  Vel-sl/1 -> Add Vel/1
  Add Accel/1 -> "dot{U}x"/1, "dot{U}y"/1, "dot{U}z"/1
  Accel-sl/1 -> Add Accel/3
  "dot{w} x r2"/1 -> Add Accel/2
  Accel-sr/1 -> "dot{w} x r2"/1
  Accel/1 -> Accel-sr/1, Accel-sl/1
  r/1 -> w x r/2, "dot{w} x r2"/2, r x 3x3/1
  "Vel-sr "/1 -> w x r/1, w x w x r/1
  w x w x r/1 -> Add Accel/1
  w x r/1 -> w x w x r/2, Add Vel/2
  Vel/1 -> "Vel-sr "/1, Vel-sl/1

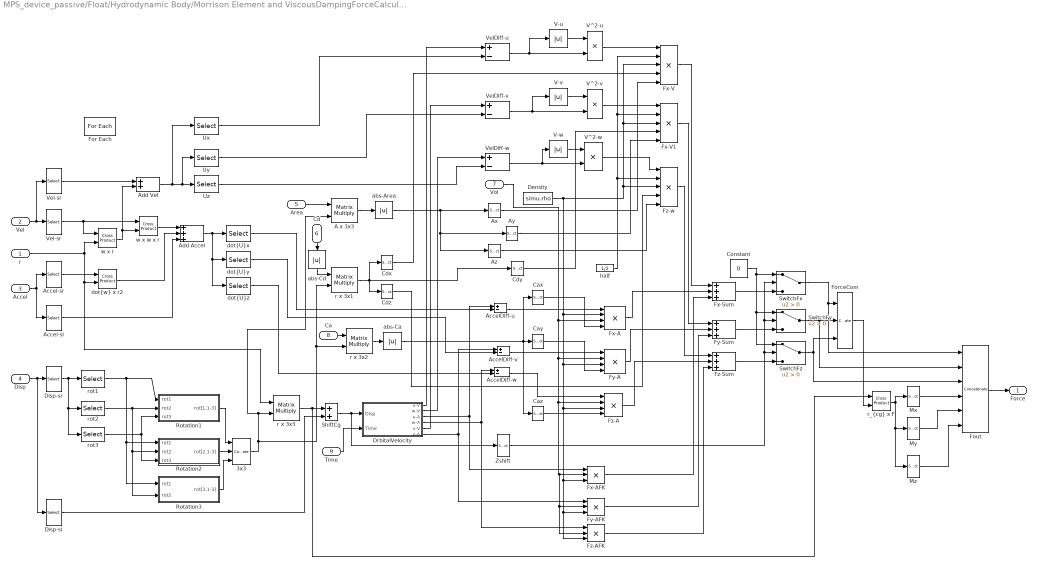
== system MPS_device_passive/Float/Hydrodynamic Body/Morrison Element and ViscousDampingForceCalculation/Morrison Element Variant Subsystem/Morrison Element On/No Wave Morison Force/MorrisonElements ==
  r : Inport  Partition=on  PartitionDimension=1  PartitionWidth=1  PartitionOffset=0
  Vel : Inport  Port=2
  Accel : Inport  Port=3
  Disp : Inport  Port=4
  Area : Inport  Port=5  Partition=on  PartitionDimension=1  PartitionWidth=1  PartitionOffset=0
  Cd : Inport  Port=6  Partition=on  PartitionDimension=1  PartitionWidth=1  PartitionOffset=0
  Vol : Inport  Port=7  Partition=on  PartitionDimension=1  PartitionWidth=1  PartitionOffset=0
  Ca : Inport  Port=8  Partition=on  PartitionDimension=1  PartitionWidth=1  PartitionOffset=0
  Time : Inport  Port=9
  3x3 : Concatenate  NumInputs=3  Mode=Multidimensional array
  A x 3x3 : Product  Multiplication=Matrix(*)
  Accel-sl : Selector  InputPortWidth=6  IndexOptions=Index vector (dialog)  Indices=[1 2 3]  OutputSizes=1
  Accel-sr : Selector  InputPortWidth=6  IndexOptions=Index vector (dialog)  Indices=[4 5 6]  OutputSizes=1
  AccelDiff-u : Sum  Inputs=+-
  AccelDiff-v : Sum  Inputs=+-
  AccelDiff-w : Sum  Inputs=+-
  Add Accel : Sum  Inputs=+++
  Add Vel : Sum
  Ax : Selector  InputPortWidth=3  IndexOptions=Index vector (dialog)  Indices=[1]  OutputSizes=1
  Ay : Selector  InputPortWidth=3  IndexOptions=Index vector (dialog)  Indices=[2]  OutputSizes=1
  Az : Selector  InputPortWidth=3  IndexOptions=Index vector (dialog)  Indices=[3]  OutputSizes=1
  Cax : Selector  InputPortWidth=3  IndexOptions=Index vector (dialog)  Indices=[1]  OutputSizes=1
  Cay : Selector  InputPortWidth=3  IndexOptions=Index vector (dialog)  Indices=[2]  OutputSizes=1
  Caz : Selector  InputPortWidth=3  IndexOptions=Index vector (dialog)  Indices=[3]  OutputSizes=1
  Cdx : Selector  InputPortWidth=3  IndexOptions=Index vector (dialog)  Indices=[1]  OutputSizes=1
  Cdy : Selector  InputPortWidth=3  IndexOptions=Index vector (dialog)  Indices=[2]  OutputSizes=1
  Cdz : Selector  InputPortWidth=3  IndexOptions=Index vector (dialog)  Indices=[3]  OutputSizes=1
  Constant : Constant  Value=0
  Density : Constant  Value=simu.rho
  Disp-sl : Selector  InputPortWidth=6  IndexOptions=Index vector (dialog)  Indices=[1 2 3]  OutputSizes=1
  Disp-sr : Selector  InputPortWidth=6  IndexOptions=Index vector (dialog)  Indices=[4 5 6]  OutputSizes=1
  For Each : ForEach  DisableCoverage=on  IndexMode=One-based
  ForceCom : Concatenate  NumInputs=3  ConcatenateDimension=2
  Fout : Concatenate  NumInputs=6  Mode=Multidimensional array  ConcatenateDimension=2
  Fx-A : Product  Inputs=4
  Fx-AFK : Product  Inputs=3
  Fx-Sum : Sum  Inputs=+++
  Fx-V : Product  Inputs=5
  Fx-V1 : Product  Inputs=5
  Fy-A : Product  Inputs=4
  Fy-AFK : Product  Inputs=3
  Fy-Sum : Sum  Inputs=+++
  Fz-A : Product  Inputs=4
  Fz-AFK : Product  Inputs=3
  Fz-Sum : Sum  Inputs=+++
  Fz-w : Product  Inputs=5
  Mx : Selector  InputPortWidth=3  IndexOptions=Index vector (dialog)  Indices=[1]  OutputSizes=1
  My : Selector  InputPortWidth=3  IndexOptions=Index vector (dialog)  Indices=[2]  OutputSizes=1
  Mz : Selector  InputPortWidth=3  IndexOptions=Index vector (dialog)  Indices=[3]  OutputSizes=1
  OrbitalVelocity : Subsystem
  Rotation1 : Subsystem
  Rotation2 : Subsystem
  Rotation3 : Subsystem
  ShiftCg : Sum
  SwitchFx : Switch  Criteria=u2 > Threshold
  SwitchFy : Switch  Criteria=u2 > Threshold
  SwitchFz : Switch  Criteria=u2 > Threshold
  Ux : Selector  InputPortWidth=3  IndexOptions=Index vector (dialog)  Indices=[1]  OutputSizes=1
  Uy : Selector  InputPortWidth=3  IndexOptions=Index vector (dialog)  Indices=[2]  OutputSizes=1
  Uz : Selector  InputPortWidth=3  IndexOptions=Index vector (dialog)  Indices=[3]  OutputSizes=1
  V-u : Abs
  V-v : Abs
  V-w : Abs
  V^2-u : Product
  V^2-v : Product
  V^2-w : Product
  Vel-sl : Selector  InputPortWidth=6  IndexOptions=Index vector (dialog)  Indices=[1 2 3]  OutputSizes=1
  "Vel-sr " : Selector  InputPortWidth=6  IndexOptions=Index vector (dialog)  Indices=[4 5 6]  OutputSizes=1
  VelDiff-u : Sum  Inputs=+-
  VelDiff-v : Sum  Inputs=+-
  VelDiff-w : Sum  Inputs=+-
  Zshift : Selector  InputPortWidth=3  IndexOptions=Index vector (dialog)  Indices=[3]  OutputSizes=1
  abs-Area : Abs
  abs-Ca : Abs
  abs-Cd : Abs
  "dot{U}x" : Selector  InputPortWidth=3  IndexOptions=Index vector (dialog)  Indices=[1]  OutputSizes=1
  "dot{U}y" : Selector  InputPortWidth=3  IndexOptions=Index vector (dialog)  Indices=[2]  OutputSizes=1
  "dot{U}z" : Selector  InputPortWidth=3  IndexOptions=Index vector (dialog)  Indices=[3]  OutputSizes=1
  "dot{w} x r2" : vrlib/Utilities/Cross Product
      settings: SourceProductBaseCode=VR
  half : Constant  Value=1/2
  r x 3x1 : Product  Multiplication=Matrix(*)
  r x 3x2 : Product  Multiplication=Matrix(*)
  r x 3x3 : Product  Multiplication=Matrix(*)
  "r_{cg} x F" : vrlib/Utilities/Cross Product
      settings: SourceProductBaseCode=VR
  rot1 : Selector  InputPortWidth=3  IndexOptions=Index vector (dialog)  Indices=[1]  OutputSizes=1
  rot2 : Selector  InputPortWidth=3  IndexOptions=Index vector (dialog)  Indices=[2]  OutputSizes=1
  rot3 : Selector  InputPortWidth=3  IndexOptions=Index vector (dialog)  Indices=[3]  OutputSizes=1
  w x r : vrlib/Utilities/Cross Product
      settings: SourceProductBaseCode=VR
  w x w x r : vrlib/Utilities/Cross Product
      settings: SourceProductBaseCode=VR
  Force : Outport  PortDimensions=[1 6]  ConcatenationDimension=1
  wires:
  Time/1 -> OrbitalVelocity/2(Time)
  abs-Cd/1 -> r x 3x1/1
  abs-Ca/1 -> Caz/1, Cay/1, Cax/1
  V-w/1 -> V^2-w/1
  Constant/1 -> SwitchFx/1, SwitchFz/1, SwitchFy/1
  Fx-V1/1 -> Fy-Sum/1
  Fy-A/1 -> Fy-Sum/2
  Cay/1 -> Fy-A/4
  AccelDiff-v/1 -> Fy-A/1
  Fy-AFK/1 -> Fy-Sum/3
  Fy-Sum/1 -> SwitchFy/3
  SwitchFy/1 -> ForceCom/2, Fout/2
  Cdy/1 -> Fx-V1/4
  Ay/1 -> Fx-V1/5
  OrbitalVelocity/5(v-V) -> VelDiff-v/1
  VelDiff-v/1 -> V^2-v/2, V-v/1
  V-v/1 -> V^2-v/1
  V^2-v/1 -> Fx-V1/1
  OrbitalVelocity/6(v-A) -> Fy-AFK/1, AccelDiff-v/1
  r x 3x2/1 -> abs-Ca/1
  Ca/1 -> r x 3x2/1
  r x 3x1/1 -> Cdx/1, Cdz/1, Cdy/1
  Cd/1 -> abs-Cd/1
  Cax/1 -> Fx-A/4
  Caz/1 -> Fz-A/4
  Fout/1 -> Force/1
  ForceCom/1 -> "r_{cg} x F"/2
  abs-Area/1 -> Ax/1, Az/1, Ay/1
  A x 3x3/1 -> abs-Area/1
  Cdz/1 -> Fz-w/4
  Cdx/1 -> Fx-V/4
  Ax/1 -> Fx-V/5
  Area/1 -> A x 3x3/1
  Az/1 -> Fz-w/5
  Fz-Sum/1 -> SwitchFz/3
  Fx-Sum/1 -> SwitchFx/3
  SwitchFx/1 -> ForceCom/1, Fout/1
  SwitchFz/1 -> Fout/3, ForceCom/3
  Zshift/1 -> SwitchFz/2, SwitchFx/2, SwitchFy/2
  VelDiff-u/1 -> V^2-u/2, V-u/1
  V-u/1 -> V^2-u/1
  3x3/1 -> r x 3x1/2, r x 3x2/2, r x 3x3/2, A x 3x3/2
  Mz/1 -> Fout/6
  My/1 -> Fout/5
  Mx/1 -> Fout/4
  "r_{cg} x F"/1 -> Mx/1, My/1, Mz/1
  Fz-AFK/1 -> Fz-Sum/3
  Fz-A/1 -> Fz-Sum/2
  Fz-w/1 -> Fz-Sum/1
  Fx-AFK/1 -> Fx-Sum/3
  Fx-A/1 -> Fx-Sum/2
  Fx-V/1 -> Fx-Sum/1
  OrbitalVelocity/4(w-A) -> AccelDiff-w/1, Fz-AFK/1
  AccelDiff-w/1 -> Fz-A/1
  Vol/1 -> Fx-A/3, Fz-A/2, Fx-AFK/2, Fz-AFK/2, Fy-AFK/2, Fy-A/2
  AccelDiff-u/1 -> Fx-A/1
  V^2-w/1 -> Fz-w/1
  Density/1 -> Fx-V/3, Fx-V1/3, Fz-w/3, Fx-A/2, Fz-A/3, Fx-AFK/3, Fz-AFK/3, Fy-AFK/3, Fy-A/3
  half/1 -> Fx-V/2, Fx-V1/2, Fz-w/2
  V^2-u/1 -> Fx-V/1
  VelDiff-w/1 -> V^2-w/2, V-w/1
  OrbitalVelocity/2(w-V) -> VelDiff-w/1
  OrbitalVelocity/1(u-V) -> VelDiff-u/1
  Uz/1 -> VelDiff-w/2
  Ux/1 -> VelDiff-u/2
  Uy/1 -> VelDiff-v/2
  Add Vel/1 -> Ux/1, Uz/1, Uy/1
  "dot{U}z"/1 -> AccelDiff-w/2
  OrbitalVelocity/3(u-A) -> Fx-AFK/1, AccelDiff-u/1
  "dot{U}x"/1 -> AccelDiff-u/2
  "dot{U}y"/1 -> AccelDiff-v/2
  ShiftCg/1 -> OrbitalVelocity/1(Disp), Zshift/1
  Disp-sl/1 -> ShiftCg/2
  r x 3x3/1 -> ShiftCg/1, "r_{cg} x F"/1
  Rotation3/1(rot[3,1-3]) -> 3x3/3
  Rotation1/1(rot[1,1-3]) -> 3x3/1
  Rotation2/1(rot[2,1-3]) -> 3x3/2
  rot2/1 -> Rotation1/2(rot2), Rotation2/2(rot2), Rotation3/2(rot2)
  rot1/1 -> Rotation1/1(rot1), Rotation2/1(rot1), Rotation3/1(rot1)
  rot3/1 -> Rotation1/3(rot3), Rotation2/3(rot3)
  Disp-sr/1 -> rot1/1, rot2/1, rot3/1
  Disp/1 -> Disp-sr/1, Disp-sl/1
  Vel-sl/1 -> Add Vel/1
  Add Accel/1 -> "dot{U}x"/1, "dot{U}y"/1, "dot{U}z"/1
  Accel-sl/1 -> Add Accel/3
  "dot{w} x r2"/1 -> Add Accel/2
  Accel-sr/1 -> "dot{w} x r2"/1
  Accel/1 -> Accel-sr/1, Accel-sl/1
  r/1 -> w x r/2, "dot{w} x r2"/2, r x 3x3/1
  "Vel-sr "/1 -> w x r/1, w x w x r/1
  w x w x r/1 -> Add Accel/1
  w x r/1 -> w x w x r/2, Add Vel/2
  Vel/1 -> "Vel-sr "/1, Vel-sl/1
